simulink model "ICCBF_RVD"  (R2024b)
settings: Solver=ode4  StartTime=0.0  StopTime=tsim  FixedStep=baseRate  RelTol=1e-6  AbsTol=1e-6
values from neighbouring files (symbols this model uses):
  a_KOZ_obs = [0.4, 0.4, 0.4]'    [Run_Initializer.m]
  a_KOZ_tar = [0.4, 0.4, 0.4]'    [Run_Initializer.m]
  a_LOS = [0.4, 0.4, 0.4]'    [Run_Initializer.m]
  beta = pi/2-atan2(docking_offset(1), docking_offset(2))    [Run_Initializer.m]
  docking_offset = [0.165 0.427 -pi/2]'    [Run_Initializer.m]
  eta = sqrt(0.5)    [Run_Initializer.m]
  f = [0 0 0 0 0 0 0]'    [Run_Initializer.m]
  gamma = (0.95)^(baseRate/t_s)    [Run_Initializer.m]
  Gamma1_el = 0.12    [Run_Initializer.m]
  Gamma1_sh = 0.005    [Run_Initializer.m]
  Gamma1_wr = 0.025    [Run_Initializer.m]
  Gamma2_el = 5    [Run_Initializer.m]
  Gamma2_sh = 5    [Run_Initializer.m]
  Gamma2_wr = 5    [Run_Initializer.m]
  Gamma3_el = 10    [Run_Initializer.m]
  Gamma3_sh = 40    [Run_Initializer.m]
  Gamma3_wr = 40    [Run_Initializer.m]
  Gamma4_el = 0.039    [Run_Initializer.m]
  Gamma4_sh = 0.015    [Run_Initializer.m]
  Gamma4_wr = 0.029    [Run_Initializer.m]
  Gamma5_el = 800    [Run_Initializer.m]
  Gamma5_sh = 800    [Run_Initializer.m]
  Gamma5_wr = 800    [Run_Initializer.m]
  Gamma6_el = 0.000001    (= 1e-06)    [Run_Initializer.m]
  Gamma6_sh = 0.005    [Run_Initializer.m]
  Gamma6_wr = 0.02    [Run_Initializer.m]
  H = 2.*diag([1 1 1 p_clf 0 0 0])    [Run_Initializer.m]
  k_dock = 5    [Run_Initializer.m]
  Kd_elarm = 0.8    [Run_Initializer.m]
  Kd_sharm = 1.0    (= 1)    [Run_Initializer.m]
  Kd_wrarm = 0.6    [Run_Initializer.m]
  Kp_elarm = 1.2    [Run_Initializer.m]
  Kp_sharm = 1.5    [Run_Initializer.m]
  Kp_wrarm = 1.0    (= 1)    [Run_Initializer.m]
  PWMFreq = 5    [Run_Initializer.m]
  Q_dock = [(lambda_dock^2)*eye(3) lambda_dock*V ... (first row only)    [Run_Initializer.m]
  r_KOZ_obs = 0.43*[1 1]'    [Run_Initializer.m]
  r_KOZ_tar_min = [0.8; 0.43]    [Run_Initializer.m]
  sensor_FOV = evalin('base', 'sensor_FOV')    [Run_Initializer.m]
  sensor_normal = evalin('base', 'sensor_normal')    [Run_Initializer.m]
  sensor_offset = evalin('base', 'sensor_offset')    [Run_Initializer.m]
  sensor_target = [0.0825 0.2516]'    [Run_Initializer.m]
  tv_CBF = 1    [Run_Initializer.m]
  Tz_lim_elarm = .1    (= 0.1)    [Run_Initializer.m]
  Tz_lim_sharm = .1    (= 0.1)    [Run_Initializer.m]
  Tz_lim_wrarm = .1    (= 0.1)    [Run_Initializer.m]
  u_max = 0.1.*[1 1 (0.3/2)-0.08]'    [Run_Initializer.m]
  x_BLACK_0 = [xLength/2 yLength/2 45*d2r 0 0 1*d2r]'    [Run_Initializer.m]
  x_BLUE_0 = [0 0 0 0 0 0]'    [Run_Initializer.m]
  zeta = 10*d2r    (= 0.174532925199)    [Run_Initializer.m]
undefined symbols (not defined in the file or in its folder): a1, a2, a3, b0, b1, b2, b3, baseRate, dataRate, delta, DiscIntNeverNeededParam, drop_states_ARM, drop_states_BLACK, drop_states_BLUE, drop_states_RED, F_red_X_nominal, F_red_Y_nominal, F_thrusters_BLACK, F_thrusters_BLUE, F_thrusters_RED, home_states_BLACK, home_states_BLUE, home_states_RED, IBLACK, IBLUE, IDIST, IEE, init_states_BLACK, init_states_BLUE, init_states_RED, IPROX, IRED, k1_KOZ_tar, k1_LOS, k2_KOZ_tar, k2_LOS, K_BLACK, K_BLUE, K_RED, k_vel, Kd_tb, Kd_tblue, Kd_tr, Kd_xb, Kd_xblue, Kd_xr, Kd_yb, Kd_yblue, Kd_yr, Kp_tb, Kp_tblue, Kp_tr, Kp_xb, Kp_xblue, Kp_xr, Kp_yb, Kp_yblue, Kp_yr, lambda_KIZ, mBLACK ... (+26)
libraries: simulink x33, nvidiaSharedBlocks x19, dspsigops x7, MainLibrary x4, dspinverses x4
(part 8 of 8)

== matlab function ICCBF_RVD/1 - Experiment Logic/Phase #3: Experiment/Sub-Phase #1/Desired Position RED/Compute Desired Position ==
  data: x_BLACK input; x_des output; docking_offset parameter
function x_des = fcn(x_BLACK, docking_offset)

R = [cos(x_BLACK(3)) -sin(x_BLACK(3)); 
     sin(x_BLACK(3))  cos(x_BLACK(3))];

r_dock = R*(docking_offset(1:2));
x_des = x_BLACK(1:3) + [r_dock; docking_offset(3)];

end

== matlab function ICCBF_RVD/3 - Control/CBF (RED)/Obstacle KOZ CBF ==
  data: x_RED input; A_KOZ_obs output; x_BLUE input; mRED parameter; r_KOZ_obs parameter; b_KOZ_obs output; a_KOZ_obs parameter; IRED parameter; platformSelection parameter
function [A_KOZ_obs, b_KOZ_obs] = fcn(x_RED, x_BLUE, mRED, r_KOZ_obs, a_KOZ_obs, IRED, platformSelection)

if platformSelection >= 6 && platformSelection <= 11
    [g_KOZ_obs, f_KOZ_obs, h_KOZ_obs] = cbf_KOZ(x_RED, x_BLUE, mRED, IRED, r_KOZ_obs, a_KOZ_obs); 
    %A_KOZ_obs = [-g_KOZ_obs, 0, 0, 0, h_KOZ_obs];
    A_KOZ_obs = [-g_KOZ_obs, 0, 0, 0, 0];
    b_KOZ_obs = f_KOZ_obs;
else
    A_KOZ_obs = [0 0 0 0 0 0 0];
    b_KOZ_obs = 0;
end

== matlab function ICCBF_RVD/3 - Control/CBF (RED)/Archives/Target KOZ CBF (OLD) ==
  data: x_RED input; A_KOZ_tar output; x_BLACK input; mRED parameter; r_KOZ_tar input; b_KOZ_tar output; k1_KOZ_tar parameter; k2_KOZ_tar parameter; tv_CBF parameter
function [A_KOZ_tar, b_KOZ_tar] = fcn(x_RED, x_BLACK, mRED, r_KOZ_tar, k1_KOZ_tar, k2_KOZ_tar, tv_CBF)

x_t = x_BLACK(1);
y_t = x_BLACK(2);
theta_t = x_BLACK(3);
x_t_dot = x_BLACK(4);
y_t_dot = x_BLACK(5);
theta_t_dot = x_BLACK(6);

x = x_RED(1);
y = x_RED(2);
x_dot = x_RED(4);
y_dot = x_RED(5);

[a,b] = deal(r_KOZ_tar(1), r_KOZ_tar(2));

A = ((cos(theta_t)/a)^2 + (sin(theta_t)/b)^2);
B = ((sin(theta_t)/a)^2 + (cos(theta_t)/b)^2);
C = 2*sin(theta_t)*cos(theta_t)*(1/a^2-1/b^2);

A_dot = theta_t_dot*sin(2*theta_t)*(b^-2 - a^-2);
B_dot = theta_t_dot*sin(2*theta_t)*(a^-2 - b^-2);
C_dot = 2*theta_t_dot*cos(2*theta_t)*(a^-2 - b^-2);

A_ddot = 2*(theta_t_dot^2)*cos(2*theta_t)*(b^-2 - a^-2);
B_ddot = 2*(theta_t_dot^2)*cos(2*theta_t)*(a^-2 - b^-2);
C_ddot = -4*(theta_t_dot^2)*sin(2*theta_t)*(a^-2 - b^-2);

Lfh = 2*A*(x-x_t)*x_dot + 2*B*(y-y_t)*y_dot + C*(x_dot*(y-y_t) + y_dot*(x-x_t));
Lf2h = 2*A*x_dot^2 + 2*B*y_dot^2 + 2*C*x_dot*y_dot;
LgLfh = [2*A*(x-x_t) + C*(y-y_t), 2*B*(y-y_t) + C*(x-x_t), 0]/mRED;

if tv_CBF == 1
    dhdt = A_dot*(x-x_t)^2 + B_dot*(y-y_t)^2 + C_dot*(x-x_t)*(y-y_t) ...
        - 2*A*(x-x_t)*x_t_dot - 2*B*(y-y_t)*y_t_dot - C*(x_t_dot*(y-y_t)+y_t_dot*(x-x_t));
    ddhddt = A_ddot*(x-x_t)^2 + B_ddot*(y-y_t)^2 + C_ddot*(x-x_t)*(y-y_t) ...
        - 4*A_dot*(x-x_t)*x_t_dot - 4*B_dot*(y-y_t)*y_t_dot ...
        - 2*C_dot*(x_t_dot*(y-y_t) + y_t_dot*(x-x_t)) + 2*A*x_t_dot^2 ...
        + 2*B*y_t_dot^2 + 2*C*x_t_dot*y_t_dot;
    ddtdhdxf = 2*A_dot*(x-x_t)*x_dot - 2*A*x_t_dot*x_dot ...
        + 2*B_dot*(y-y_t)*y_dot - 2*B*y_t_dot*y_dot ...
        + C_dot*(x_dot*(y-y_t) + y_dot*(x-x_t)) - C*(x_t_dot*y_dot + y_t_dot*x_dot);
else
    dhdt = 0;
    ddhddt = 0;
    ddtdhdxf = 0;
end

h = A*(x-x_t)^2 + B*(y-y_t)^2 + C*(x-x_t)*(y-y_t)-1;
h_dot = Lfh + dhdt;

A_KOZ_tar = [-LgLfh 0];
b_KOZ_tar = Lf2h + 2*ddtdhdxf + ddhddt + 2*sqrt(k1_KOZ_tar)*k2_KOZ_tar*h_dot + k1_KOZ_tar*h;

end

== matlab function ICCBF_RVD/3 - Control/CBF (RED)/Archives/Nominal LQR Controller/Calculate Error/MATLAB Function ==
  data: Rz_path input; Rz_error output; Rz_measured input
function Rz_error = SmoothAngularDifference(Rz_path, Rz_measured)

    Rz_error = mod(Rz_measured-Rz_path+pi, 2*pi)-pi;


end

== matlab function ICCBF_RVD/3 - Control/CBF (RED)/Apply CBFs ==
  data: u output; x output; A_KOZ_tar input; b_KOZ_tar input; A_LOS input; b_LOS input; A_KOZ_obs input; b_KOZ_obs input; res output; A_dock input; b_dock input; x0 input; u_max parameter; H parameter; f parameter
function [u, x, res] = fcn(A_KOZ_tar, b_KOZ_tar, A_LOS, b_LOS, A_KOZ_obs, b_KOZ_obs, A_dock, b_dock, x0, u_max, H, f)

A = [A_KOZ_tar; A_LOS; A_KOZ_obs; A_dock];
b = [b_KOZ_tar; b_LOS; b_KOZ_obs; b_dock];

options = optimoptions('quadprog', 'Algorithm', 'active-set', 'MaxIterations', 20);

tic
[x, ~, exitflag, output] = quadprog(H, f, A, b, [], [], [-u_max; 0; 0; 0; 0], [u_max; inf; inf; inf; inf], x0, options);
res = [double(exitflag), double(output.iterations), toc];

u = x(1:3);

end

== matlab function ICCBF_RVD/3 - Control/CBF (RED)/Archives/Velocity CBF (OLD) ==
  data: x_RED input; A_vel output; b_vel output; mRED parameter; k_vel parameter; v_max parameter
function [A_vel, b_vel] = fcn(x_RED, mRED, k_vel, v_max)

x_dot = x_RED(4);
y_dot = x_RED(5);

v_mag = sqrt(x_dot^2+y_dot^2);

Lgh = [(-x_dot/(mRED*v_mag)) (-y_dot/(mRED*v_mag)) 0];
   
h = v_max-v_mag;

A_vel = -Lgh;
b_vel = k_vel*h;

end

== matlab function ICCBF_RVD/Simulate Plant Dynamics/RED and ARM Dynamics/RED Only/Calculated & Store Measured States/Subsystem1/Enabled Subsystem/MATLAB Function ==
  data: y input; dy output; dt input; tau input; ema_prev input; ema output
function [dy, ema] = realtime_derivative_ema(y, dt, tau, ema_prev)
    % Compute smoothed derivative using Exponential Moving Average
    %
    % Inputs:
    %   y        : Current measurement
    %   dt       : Time step
    %   tau      : Time constant for EMA filter (larger = more smoothing)
    %   ema_prev : Previous EMA value
    %
    % Outputs:
    %   dy  : Smoothed derivative estimate
    %   ema : Updated EMA value
    
    % Calculate smoothing factor from time constant
    alpha = 1 - exp(-dt ./ tau);
    
    % Update Exponential Moving Average
    ema = alpha .* y + (1 - alpha) .* ema_prev;
    
    % Compute derivative using finite difference on smoothed values
    dy = (ema - ema_prev) ./ dt;
end

== matlab function ICCBF_RVD/3 - Control/CBF (RED)/Archives/Build Table KIZ CBF ==
  data: x_RED input; A output; b output; delta parameter; mRED parameter; xLength parameter; yLength parameter; lambda_KIZ parameter
function [A, b] = fcn(x_RED, delta, mRED, xLength, yLength, lambda_KIZ)

x = x_RED(1);
x_dot = x_RED(4);

y = x_RED(2);
y_dot = x_RED(5);

h_upper_x = x-delta;
h_dot_upper_x = x_dot;

h_lower_x = -x-delta+xLength;
h_dot_lower_x = -x_dot;

A_upper_x = [-1/mRED 0 0];
b_upper_x = (lambda_KIZ^2)*h_upper_x + 2*lambda_KIZ*h_dot_upper_x;

A_lower_x = [1/mRED 0 0];
b_lower_x = (lambda_KIZ^2)*h_lower_x + 2*lambda_KIZ*h_dot_lower_x;

h_upper_y = y-delta;
h_dot_upper_y = y_dot;

h_lower_y = -y-delta+yLength;
h_dot_lower_y = -y_dot;

A_upper_y = [0 -1/mRED 0];
b_upper_y = (lambda_KIZ^2)*h_upper_y + 2*lambda_KIZ*h_dot_upper_y;

A_lower_y = [0 1/mRED 0];
b_lower_y = (lambda_KIZ^2)*h_lower_y + 2*lambda_KIZ*h_dot_lower_y;

A = [A_upper_x; A_lower_x; A_upper_y; A_lower_y];
b = [b_upper_x; b_lower_x; b_upper_y; b_lower_y];

end

== matlab function ICCBF_RVD/Thruster & Float Control Code/Change BLACK Behavior/Calculate Duty Cycle/Generate Initial Guess/MATLAB Function ==
  data: H output; thruster_dist2CG_BLACK parameter; F_thrusters_BLACK parameter
function H = MakeH(thruster_dist2CG_BLACK,F_thrusters_BLACK)

    Vec1 = [ -1
             -1
              0 
              0
              1
              1
              0
              0 ];
          
    Vec2 = [  0
              0
              1
              1
              0
              0
             -1
             -1 ];
         
    Vec3 = thruster_dist2CG_BLACK./1000;
    
    Mat1 = [Vec1, Vec2, Vec3]';
    
    Mat2 = diag((F_thrusters_BLACK./2));
    
    H    = Mat1*Mat2;

end

== matlab function ICCBF_RVD/Thruster & Float Control Code/Change RED Behavior/Calculate Duty Cycle/MATLAB Function5 ==
  data: H_final output; u_desired input; duty_cycles output; x0 input; thruster_dist2CG_RED parameter; F_red_X_nominal parameter; F_red_Y_nominal parameter; max_iters parameter; tol parameter
function [H_final, duty_cycles] = optimize_duty_cycle_with_decay( ...
    u_desired, x0, thruster_dist2CG_RED, F_red_X_nominal, F_red_Y_nominal, max_iters, tol)
    %OPTIMIZE_DUTY_CYCLE_WITH_DECAY 
    %   Iteratively optimizes thruster duty cycles while updating thrust decay.
    %
    %   Inputs:
    %       u_desired           - Desired force/torque vector [Fx; Fy; M] (3x1)
    %       x0                  - Initial guess for duty cycles (8x1)
    %       thruster_dist2CG_RED- Distances of thrusters from CG (vector, mm)
    %       F_red_X_nominal     - Nominal X-direction thruster force (scalar, N)
    %       F_red_Y_nominal     - Nominal Y-direction thruster force (scalar, N)
    %       max_iters           - Maximum optimization iterations
    %       tol                 - Convergence tolerance (on duty cycles)
    %
    %   Outputs:
    %       H_final     - Final H-matrix including thrust decay (3x8)
    %       duty_cycles - Optimized duty cycles (8x1)
    %

    % ---------------------------
    % Initialization
    % ---------------------------
    num_thrusters      = length(x0); %#ok<NASGU> % reserved if needed later
    duty_cycles        = x0;                     % current solution
    thrust_decay_factor = 1;                     % initial decay
    prev_duty_cycles   = duty_cycles + 2*tol;    % force first iteration

    % ---------------------------
    % Iterative optimization
    % ---------------------------
    for iter = 1:max_iters
        % Build system matrix H with current decay factor
        H = MakeHWithDecay(thruster_dist2CG_RED, F_red_X_nominal, ...
                           thrust_decay_factor, F_red_Y_nominal);

        % Solve constrained least squares (box constraints: 0 ≤ x ≤ 1)
        duty_cycles = custom_constrained_least_squares(H, u_desired, duty_cycles);

        % Update decay factor based on the current duty cycles
        [thrust_decay_factor, ~] = check_thrust_decay(duty_cycles);

        % Check convergence (∞-norm difference)
        if norm(duty_cycles - prev_duty_cycles, Inf) < tol
            H_final = MakeHWithDecayRecalculateForce(thruster_dist2CG_RED, ...
                        F_red_X_nominal, thrust_decay_factor, F_red_Y_nominal);
            return;
        end

        % Update reference for next iteration
        prev_duty_cycles = duty_cycles;
    end

    % If not converged within max_iters, return final H with last decay
    H_final = MakeHWithDecayRecalculateForce(thruster_dist2CG_RED, ...
                F_red_X_nominal, thrust_decay_factor, F_red_Y_nominal);
end


% ========================================================================
% Custom Constrained Least Squares Solver
% ========================================================================
function x_opt = custom_constrained_least_squares(H, b, x0)
    %CUSTOM_CONSTRAINED_LEAST_SQUARES
    %   Solves min_x ||H*x - b||^2 subject to 0 <= x <= 1
    %   using projected gradient descent with backtracking line search.
    %
    %   Inputs:
    %       H   - System matrix (3x8)
    %       b   - Desired vector (3x1)
    %       x0  - Initial guess (8x1)
    %
    %   Output:
    %       x_opt - Optimal duty cycle vector (8x1)

    % Parameters
    max_iterations = 100;
    tolerance      = 1e-6;
    alpha          = 0.01;  % initial step size
    beta           = 0.5;   % backtracking factor

    % Initialization
    x      = x0;
    x_prev = x0 + 2*tolerance;

    % Precompute matrices
    HtH = H' * H;
    Htb = H' * b;

    for iter = 1:max_iterations
        % Gradient of ||H*x - b||^2
        gradient = 2 * (HtH*x - Htb);

        % Store objective for comparison
        current_obj = norm(H*x - b)^2;

        % Backtracking line search
        step_size = alpha;
        for ls_iter = 1:20
            x_new = x - step_size * gradient;
            x_new = max(0, min(1, x_new)); % project into [0,1]

            new_obj = norm(H*x_new - b)^2;
            if new_obj < current_obj
                break; % accept step
            else
                step_size = step_size * beta;
            end
        end

        % Update
        x = x_new;

        % Convergence check
        if norm(x - x_prev) < tolerance
            break;
        end

        % Adaptive step size tuning
        if iter > 1 && new_obj < current_obj
            alpha = min(alpha * 1.1, 0.1); % speed up if progress
        else
            alpha = alpha * 0.9;           % slow down otherwise
        end

        % Store for next iteration
        x_prev = x;
    end

    x_opt = x;
end


% ========================================================================
% Construct H-matrix (with decay factor)
% ========================================================================
function H = MakeHWithDecay(thruster_dist2CG, F_X_nominal, thrust_decay_factor, F_Y_nominal)
    %MAKEHWITHDECAY
    %   Builds the H matrix that maps thruster duty cycles to [Fx; Fy; M],
    %   applying thrust decay.
    %
    %   Outputs H as (3x8)

    % Convert thruster arm distances to meters
    adjusted_dist = thruster_dist2CG / 1000;

    % Thruster directions (X, Y, and moment arm)
    Vec1 = [-1; -1;  0;  0;  1;  1;  0;  0]; % X
    Vec2 = [ 0;  0;  1;  1;  0;  0; -1; -1]; % Y
    Vec3 = adjusted_dist;                    % moment (Z)

    Mat1 = [Vec1, Vec2, Vec3]';

    % Thruster forces (scaled by decay)
    F_thrusters = [F_X_nominal; F_X_nominal; ...
                   F_Y_nominal; F_Y_nominal; ...
                   F_X_nominal; F_X_nominal; ...
                   F_Y_nominal; F_Y_nominal] * thrust_decay_factor;

    % Build diagonal scaling
    Mat2 = diag(F_thrusters / 2);

    % Final mapping
    H = Mat1 * Mat2;
end


% ========================================================================
% Construct H-matrix (recalculate full force with decay)
% ========================================================================
function H = MakeHWithDecayRecalculateForce(thruster_dist2CG, F_X_nominal, thrust_decay_factor, F_Y_nominal)
    %MAKEHWITHDECAYRECALCULATEFORCE
    %   Same as MakeHWithDecay but applies full nominal force scaling.

    adjusted_dist = thruster_dist2CG / 1000;

    Vec1 = [-1; -1;  0;  0;  1;  1;  0;  0];
    Vec2 = [ 0;  0;  1;  1;  0;  0; -1; -1];
    Vec3 = adjusted_dist;

    Mat1 = [Vec1, Vec2, Vec3]';

    F_thrusters = [F_X_nominal; F_X_nominal; ...
                   F_Y_nominal; F_Y_nominal; ...
                   F_X_nominal; F_X_nominal; ...
                   F_Y_nominal; F_Y_nominal] * thrust_decay_factor;

    Mat2 = diag(F_thrusters);

    H = Mat1 * Mat2;
end


% ========================================================================
% Thrust Decay Update Rule
% ========================================================================
function [thrust_decay_factor, count] = check_thrust_decay(PWMs)
    %CHECK_THRUST_DECAY
    %   Updates thrust decay factor based on average duty cycle.
    %
    %   Inputs:
    %       PWMs - Duty cycle vector (8x1)
    %
    %   Outputs:
    %       thrust_decay_factor - Adjusted decay factor (scalar)
    %       count               - Number of active thrusters

    % Normalize if needed
    if max(PWMs) > 1
        PWMs = PWMs / max(PWMs);
    end
    
    % Active thrusters
    count = sum(PWMs > 0);
    
    % Mean duty cycle (only active thrusters)
    avg_duty = sum(max(PWMs, 0)) / max(count, 1);
    
    % Update rule (piecewise)
    if avg_duty < 0.3 || count == 0
        thrust_decay_factor = 1;
    else
        thrust_decay_factor = max(0.6 - 2*avg_duty + 1, 0.5);
    end
end

== matlab function ICCBF_RVD/Thruster & Float Control Code/Change BLACK Behavior/Calculate Duty Cycle/Rotate Forces to Inertial/Create Rotation Matrix ==
  data: Rz input; C_Ib output
function C_Ib = RotateFrame(Rz)

C_bI = [  cos(Rz) sin(Rz)
         -sin(Rz) cos(Rz) ];

C_Ib = inv(C_bI);

end

== matlab function ICCBF_RVD/3 - Control/CBF (RED)/Docking CLF ==
  data: x_RED input; x_BLACK input; A_dock output; b_dock output; mRED parameter; IRED parameter; docking_offset parameter; Q_dock parameter; k_dock parameter; tv_CBF parameter
function [A_dock, b_dock] = fcn(x_RED, x_BLACK, mRED, IRED, docking_offset, Q_dock, k_dock, tv_CBF)

B = [  0       0      0;
       0       0      0;
       0       0      0;
     1/mRED    0      0;
     0      1/mRED    0;
     0         0   1/IRED];

R = [cos(x_BLACK(3)) -sin(x_BLACK(3)); 
     sin(x_BLACK(3))  cos(x_BLACK(3))];
dR = [-sin(x_BLACK(3)) -cos(x_BLACK(3)); 
       cos(x_BLACK(3))  -sin(x_BLACK(3))];

r_des = x_BLACK(1:2) + R*(docking_offset(1:2));
theta_des = wrapAngle(x_BLACK(3) + docking_offset(3));
v_des = x_BLACK(4:5) + x_BLACK(6)*dR*(docking_offset(1:2));
omega_des = x_BLACK(6);

x_des = [r_des; theta_des; v_des; omega_des];

LfV = 2*(x_RED-x_des)'*Q_dock*[x_RED(4:6); 0; 0; 0];
LgV = 2*(x_RED-x_des)'*Q_dock*B;

if tv_CBF == 1
    dVdt = -2*(x_RED-x_des)'*Q_dock*[x_des(4:6); 0; 0; 0];
else
    dVdt = 0;
end

A_dock = [LgV -1 0 0 0];
b_dock = (-LfV - dVdt - k_dock*(x_RED-x_des)'*Q_dock*(x_RED-x_des)); 

end

%% Functions

function theta_wrap = wrapAngle(theta)
    theta_wrap = atan2(sin(theta),cos(theta));
end

== matlab function ICCBF_RVD/Thruster & Float Control Code/Change RED Behavior/Calculate Duty Cycle/MATLAB Function8 ==
  data: ThrustPer_Final output; ThrustPer input; PWMFreq parameter
function ThrustPer_Final  = ThrusterSat(ThrustPer, PWMFreq)

    ValveTime       = 0.007;
    TControl        = 1/PWMFreq;

    ThrustPer_Final = zeros(8,1);
    
    if max(ThrustPer) > 1
        ThrustPer_Sat = ThrustPer/max(ThrustPer);
    else
        ThrustPer_Sat = ThrustPer;
    end
    
    for i = 1:8
        if ThrustPer_Sat(i) > ValveTime/TControl 
            ThrustPer_Final(i) = ThrustPer_Sat(i);
        else
            ThrustPer_Final(i) = 0;
        end
    end


end

== matlab function ICCBF_RVD/Thruster & Float Control Code/Change BLACK Behavior/Rotate Forces to Body/Create Rotation Matrix ==
  data: Rz input; C_bI output
function C_bI = RotateFrame(Rz)

C_bI = [  cos(Rz) sin(Rz)
         -sin(Rz) cos(Rz) ];

end

== matlab function ICCBF_RVD/3 - Control/CBF (RED)/Archives/LOS CBF original (OLD) ==
  data: x_RED input; A_LOS output; x_BLACK input; b_LOS output; k2_LOS parameter; k1_LOS parameter; theta_FOV parameter; IRED parameter; tv_CBF parameter
function [A_LOS, b_LOS] = fcn(x_RED, x_BLACK, k2_LOS, k1_LOS, theta_FOV, IRED, tv_CBF)

x_t = x_BLACK(1);
y_t = x_BLACK(2);
x_t_dot = x_BLACK(4);
y_t_dot = x_BLACK(5);

x = x_RED(1);
y = x_RED(2);
theta = x_RED(3);
x_dot = x_RED(4);
y_dot = x_RED(5);
theta_dot = x_RED(6);
x_ddot = 0;
y_ddot = 0;

theta_star = rotateToFace(x_RED(3), x_BLACK(1:2)-x_RED(1:2));

rmagsq = (x_t-x)^2+(y_t-y)^2;
drmagsqdt = 2*(x_t-x)*(x_t_dot-x_dot)+2*(y_t-y)*(y_t_dot-y_dot);

Lfh = -theta_dot;
LgLfh = [0, 0, -1/IRED];

if tv_CBF == 1
    dh_dt = -((x_t_dot-x_dot)*(y_t-y)-(y_t_dot-y_dot)*(x_t-x))/(rmagsq);
    ddh_dtt = (((y_ddot*(x_t-x)-x_ddot*(y_t-y))*rmagsq) - drmagsqdt*((x_t_dot-x_dot)*(y_t-y)-(y_t_dot-y_dot)*(x_t-x)))/rmagsq^2;
    ddtdhdxf = 0;    
else
    dh_dt = 0;
    ddh_dtt = 0;
    ddtdhdxf = 0;    
end

h_upper = -theta + theta_star + theta_FOV;
h_lower = theta - theta_star + theta_FOV;

h_dot_upper = Lfh + dh_dt;
h_dot_lower = -Lfh - dh_dt;

A_upper = -LgLfh;
A_lower = -(-LgLfh);

b_upper = -2*ddtdhdxf + ddh_dtt + 2*sqrt(k1_LOS)*k2_LOS*h_dot_upper + k1_LOS*h_upper;
b_lower = (-2*ddtdhdxf) + (-ddh_dtt) + 2*sqrt(k1_LOS)*k2_LOS*h_dot_lower + k1_LOS*h_lower;

A_LOS = [A_lower; A_upper];
b_LOS = [b_lower; b_upper];

end

%% Functions

function theta_des = rotateToFace(theta, r)
    theta_des = theta + wrapToPi(atan2(r(2),r(1)) - theta);
end

== matlab function ICCBF_RVD/Thruster & Float Control Code/Change BLUE Behavior/Calculate Duty Cycle/Generate Initial Guess/MATLAB Function ==
  data: H output; thruster_dist2CG_BLUE parameter; F_thrusters_BLUE parameter
function H = MakeH(thruster_dist2CG_BLUE,F_thrusters_BLUE)

    Vec1 = [ -1
             -1
              0 
              0
              1
              1
              0
              0 ];
          
    Vec2 = [  0
              0
              1
              1
              0
              0
             -1
             -1 ];
         
    Vec3 = thruster_dist2CG_BLUE./1000;
    
    Mat1 = [Vec1, Vec2, Vec3]';
    
    Mat2 = diag((F_thrusters_BLUE./2));
    
    H    = Mat1*Mat2;

end

== matlab function ICCBF_RVD/3 - Control/CBF (RED)/Archives/LOS CBF alt (OLD) ==
  data: x_RED input; A_LOS output; x_BLACK input; b_LOS output; k2_LOS parameter; k1_LOS parameter; theta_FOV parameter; IRED parameter; tv_CBF parameter
function [A_LOS, b_LOS] = fcn(x_RED, x_BLACK, k2_LOS, k1_LOS, theta_FOV, IRED, tv_CBF)

x_t = x_BLACK(1);
y_t = x_BLACK(2);
x_t_dot = x_BLACK(4);
y_t_dot = x_BLACK(5);

x = x_RED(1);
y = x_RED(2);
theta = x_RED(3);
theta_dot = x_RED(6);

theta_star = rotateToFace(x_RED(3), x_BLACK(1:2)-x_RED(1:2));

rmagsq = (x_t-x)^2+(y_t-y)^2;

Lfh = -theta_dot;

LgLfh = [0, 0, -1/IRED];

dthetastar_dt = (y_t_dot*(x_t-x) - x_t_dot*(y_t-y))/(rmagsq);
ddthetastar_dt = -2*(((x_t-x)*y_t_dot - (y_t-y)*x_t_dot)*((x_t-x)*x_t_dot+(y_t-y)*y_t_dot))/rmagsq^2;
if tv_CBF == 1
    dh_dt = dthetastar_dt;
    ddh_dtt = ddthetastar_dt;
    ddtdhdxf = 0;    
else
    dh_dt = 0;
    ddh_dtt = 0;
    ddtdhdxf = 0;    
end

h_upper = -theta + theta_star + theta_FOV;
h_lower = theta - theta_star + theta_FOV;

h_dot_upper = Lfh + dh_dt;
h_dot_lower = -Lfh - dh_dt;

A_upper = -LgLfh;
A_lower = -(-LgLfh);

b_upper =  2*ddtdhdxf + ddh_dtt + 2*sqrt(k1_LOS)*k2_LOS*h_dot_upper + k1_LOS*h_upper;
b_lower = (-2*ddtdhdxf) + (-ddh_dtt) + 2*sqrt(k1_LOS)*k2_LOS*h_dot_lower + k1_LOS*h_lower;

A_LOS = [A_lower; A_upper];
b_LOS = [b_lower; b_upper];

end

%% Functions

function theta_des = rotateToFace(theta, r)
    theta_des = theta + wrapToPi(atan2(r(2),r(1)) - theta);
end

== matlab function ICCBF_RVD/Thruster & Float Control Code/Change BLUE Behavior/Calculate Duty Cycle/MATLAB Function1 ==
  data: ThrustPer_Final output; ThrustPer input; PWMFreq parameter
function ThrustPer_Final  = ThrusterSat(ThrustPer, PWMFreq)

    ValveTime       = 0.007;
    TControl        = 1/PWMFreq;

    ThrustPer_Final = zeros(8,1);
    
    if max(ThrustPer) > 1
        ThrustPer_Sat = ThrustPer/max(ThrustPer);
    else
        ThrustPer_Sat = ThrustPer;
    end
    
    for i = 1:8
        if ThrustPer_Sat(i) > ValveTime/TControl 
            ThrustPer_Final(i) = ThrustPer_Sat(i);
        else
            ThrustPer_Final(i) = 0;
        end
    end


end

== matlab function ICCBF_RVD/Thruster & Float Control Code/Change BLUE Behavior/Calculate Duty Cycle/Rotate Forces to Inertial/Create Rotation Matrix ==
  data: Rz input; C_Ib output
function C_Ib = RotateFrame(Rz)

C_bI = [  cos(Rz) sin(Rz)
         -sin(Rz) cos(Rz) ];

C_Ib = inv(C_bI);

end

== matlab function ICCBF_RVD/Thruster & Float Control Code/Change RED Behavior/Calculate Duty Cycle/Rotate Forces to Inertial/Create Rotation Matrix ==
  data: Rz input; C_Ib output
function C_Ib = RotateFrame(Rz)

C_bI = [  cos(Rz) sin(Rz)
         -sin(Rz) cos(Rz) ];

C_Ib = inv(C_bI);

end

== matlab function ICCBF_RVD/Thruster & Float Control Code/Change BLUE Behavior/Rotate Forces to Body/Create Rotation Matrix ==
  data: Rz input; C_bI output
function C_bI = RotateFrame(Rz)

C_bI = [  cos(Rz) sin(Rz)
         -sin(Rz) cos(Rz) ];

end

== matlab function ICCBF_RVD/1 - Experiment Logic/Phase #3: Experiment/Sub-Phase #2/Desired Position BLACK/Safe Desired Position ==
  data: x_des input; x_des output; x_des_prev input; xLength parameter; yLength parameter
function x_des = fcn(x_des,x_des_prev, xLength, yLength)

corners = [0 0;
           xLength 0;
           xLength yLength;
           0 yLength];

walls = [ 1  0;
          0  1;
         -1  0;
          0 -1];

edge = 0;
for j = 1:length(walls)
    wall_normal = [-walls(j,2); walls(j,1)];

    if dot(x_des(4:5), -wall_normal) > 0
        % Not moving towards wall
        continue
    end

    d = norm(dot(x_des(1:2) - corners(j,:)', wall_normal))/norm(walls(j,:)');
    if d <= 0.3
        edge = 1;
        break
    end
end

if edge
    x_des = x_des_prev;
end

== matlab function ICCBF_RVD/1 - Experiment Logic/Phase #3: Experiment/Sub-Phase #2/Desired Position BLUE/Safe Desired Position ==
  data: x_des input; x_des output; x_des_prev input; xLength parameter; yLength parameter
function x_des = fcn(x_des,x_des_prev, xLength, yLength)

corners = [0 0;
           xLength 0;
           xLength yLength;
           0 yLength];

walls = [ 1  0;
          0  1;
         -1  0;
          0 -1];

edge = 0;
for j = 1:length(walls)
    wall_normal = [-walls(j,2); walls(j,1)];

    if dot(x_des(4:5), -wall_normal) > 0
        % Not moving towards wall
        continue
    end

    d = norm(dot(x_des(1:2) - corners(j,:)', wall_normal))/norm(walls(j,:)');
    if d <= 0.3
        edge = 1;
        break
    end
end

if edge
    x_des = x_des_prev;
end

== matlab function ICCBF_RVD/3 - Control/CBF (RED)/Target KOZ ICCBF ==
  data: x_RED input; A_KOZ_tar output; x_BLACK input; mRED parameter; IRED parameter; b_KOZ_tar output; a_KOZ_tar parameter; r_KOZ_tar input
function [A_KOZ_tar, b_KOZ_tar] = fcn(x_RED, x_BLACK, mRED, IRED, a_KOZ_tar, r_KOZ_tar)

[g_KOZ_tar, f_KOZ_tar, h_KOZ_tar] = cbf_KOZ(x_RED, x_BLACK, mRED, IRED, r_KOZ_tar, a_KOZ_tar);

%A_KOZ_tar = [-g_KOZ_tar, 0, h_KOZ_tar, 0, 0];
A_KOZ_tar = [-g_KOZ_tar, 0, 0, 0, 0];
b_KOZ_tar = f_KOZ_tar;

end

== matlab function ICCBF_RVD/Thruster & Float Control Code/Change RED Behavior/Rotate Forces to Body/Create Rotation Matrix ==
  data: Rz input; C_bI output
function C_bI = RotateFrame(Rz)

C_bI = [  cos(Rz) sin(Rz)
         -sin(Rz) cos(Rz) ];

end

== matlab function ICCBF_RVD/1 - Experiment Logic/Phase #3: Experiment/Sub-Phase #2/Desired Position RED/Compute Desired Position ==
  data: x_BLACK input; x_des output; docking_offset parameter
function x_des = fcn(x_BLACK, docking_offset)

R = [cos(x_BLACK(3)) -sin(x_BLACK(3)); 
     sin(x_BLACK(3))  cos(x_BLACK(3))];

r_dock = R*(docking_offset(1:2));
x_des = x_BLACK(1:3) + [r_dock; docking_offset(3)];

end

== matlab function ICCBF_RVD/3 - Control/CBF (RED)/Clamp to u_max ==
  data: u input; u output; u_max parameter
function u = fcn(u, u_max)

if abs(u(1)) > u_max(1)
    u(1) = sign(u(1))*u_max(1);
end 

if abs(u(2)) > u_max(2)
    u(2) = sign(u(2))*u_max(2);
end 

if abs(u(3)) > u_max(3)
    u(3) = sign(u(3))*u_max(3);
end

end

== matlab function ICCBF_RVD/3 - Control/Default LQR Control (RED)/Calculate Error/MATLAB Function ==
  data: Rz_path input; Rz_error output; Rz_measured input
function Rz_error = SmoothAngularDifference(Rz_path, Rz_measured)

    Rz_error = mod(Rz_measured-Rz_path+pi, 2*pi)-pi;


end

== matlab function ICCBF_RVD/1 - Experiment Logic/Phase #3: Experiment/Sub-Phase #1/Desired Position BLUE/Safe Desired Position ==
  data: x_des input; x_des output; x_des_prev input; xLength parameter; yLength parameter
function x_des = fcn(x_des,x_des_prev, xLength, yLength)

corners = [0 0;
           xLength 0;
           xLength yLength;
           0 yLength];

walls = [ 1  0;
          0  1;
         -1  0;
          0 -1];

edge = 0;
for j = 1:length(walls)
    wall_normal = [-walls(j,2); walls(j,1)];

    if dot(x_des(1:2)-x_des_prev(1:2), wall_normal) > 0
        % Not moving towards wall
        continue
    end

    d = norm(dot(x_des(1:2) - corners(j,:)', wall_normal))/norm(walls(j,:)');
    if d <= 0.3
        edge = 1;
        break
    end
end

if edge
    x_des = x_des_prev;
end

== matlab function ICCBF_RVD/1 - Experiment Logic/Phase #3: Experiment/Sub-Phase #1/Desired Position BLACK/Safe Desired Position ==
  data: x_des input; x_des output; x_des_prev input; xLength parameter; yLength parameter
function x_des = fcn(x_des,x_des_prev, xLength, yLength)

corners = [0 0;
           xLength 0;
           xLength yLength;
           0 yLength];

walls = [ 1  0;
          0  1;
         -1  0;
          0 -1];

edge = 0;
for j = 1:length(walls)
    wall_normal = [-walls(j,2); walls(j,1)];

    if dot(x_des(1:2)-x_des_prev(1:2), wall_normal) > 0
        % Not moving towards wall
        continue
    end

    d = norm(dot(x_des(1:2) - corners(j,:)', wall_normal))/norm(walls(j,:)');
    if d <= 0.3
        edge = 1;
        break
    end
end

if edge
    x_des = x_des_prev;
end

== matlab function ICCBF_RVD/1 - Experiment Logic/Phase #3: Experiment/Sub-Phase #3/Desired Position BLACK/Safe Desired Position ==
  data: x_des input; x_des output; x_des_prev input; xLength parameter; yLength parameter
function x_des = fcn(x_des,x_des_prev, xLength, yLength)

corners = [0 0;
           xLength 0;
           xLength yLength;
           0 yLength];

walls = [ 1  0;
          0  1;
         -1  0;
          0 -1];

edge = 0;
for j = 1:length(walls)
    wall_normal = [-walls(j,2); walls(j,1)];

    if dot(x_des(4:5), -wall_normal) > 0
        % Not moving towards wall
        continue
    end

    d = norm(dot(x_des(1:2) - corners(j,:)', wall_normal))/norm(walls(j,:)');
    if d <= 0.3
        edge = 1;
        break
    end
end

if edge
    x_des = x_des_prev;
end

== matlab function ICCBF_RVD/1 - Experiment Logic/Phase #3: Experiment/Sub-Phase #3/Desired Position BLUE/Safe Desired Position ==
  data: x_des input; x_des output; x_des_prev input; xLength parameter; yLength parameter
function x_des = fcn(x_des,x_des_prev, xLength, yLength)

corners = [0 0;
           xLength 0;
           xLength yLength;
           0 yLength];

walls = [ 1  0;
          0  1;
         -1  0;
          0 -1];

edge = 0;
for j = 1:length(walls)
    wall_normal = [-walls(j,2); walls(j,1)];

    if dot(x_des(4:5), -wall_normal) > 0
        % Not moving towards wall
        continue
    end

    d = norm(dot(x_des(1:2) - corners(j,:)', wall_normal))/norm(walls(j,:)');
    if d <= 0.3
        edge = 1;
        break
    end
end

if edge
    x_des = x_des_prev;
end

== matlab function ICCBF_RVD/1 - Experiment Logic/Phase #3: Experiment/Sub-Phase #3/Desired Position RED/Compute Desired Position ==
  data: x_BLACK input; x_des output; docking_offset parameter
function x_des = fcn(x_BLACK, docking_offset)

R = [cos(x_BLACK(3)) -sin(x_BLACK(3)); 
     sin(x_BLACK(3))  cos(x_BLACK(3))];

r_dock = R*(docking_offset(1:2));
x_des = x_BLACK(1:3) + [r_dock; docking_offset(3)];

end

== matlab function ICCBF_RVD/Thruster & Float Control Code/Change BLACK Behavior/Calculate Duty Cycle/MATLAB Function1 ==
  data: ThrustPer_Final output; ThrustPer input; PWMFreq parameter
function ThrustPer_Final  = ThrusterSat(ThrustPer, PWMFreq)

    ValveTime       = 0.007;
    TControl        = 1/PWMFreq;

    ThrustPer_Final = zeros(8,1);
    
    if max(ThrustPer) > 1
        ThrustPer_Sat = ThrustPer/max(ThrustPer);
    else
        ThrustPer_Sat = ThrustPer;
    end
    
    for i = 1:8
        if ThrustPer_Sat(i) > ValveTime/TControl 
            ThrustPer_Final(i) = ThrustPer_Sat(i);
        else
            ThrustPer_Final(i) = 0;
        end
    end


end

== matlab function ICCBF_RVD/1 - Experiment Logic/Phase #3: Experiment/Sub-Phase #4/Desired Position BLACK/Safe Desired Position ==
  data: x_des input; x_des output; x_des_prev input; xLength parameter; yLength parameter
function x_des = fcn(x_des,x_des_prev, xLength, yLength)

corners = [0 0;
           xLength 0;
           xLength yLength;
           0 yLength];

walls = [ 1  0;
          0  1;
         -1  0;
          0 -1];

edge = 0;
for j = 1:length(walls)
    wall_normal = [-walls(j,2); walls(j,1)];

    if dot(x_des(4:5), -wall_normal) > 0
        % Not moving towards wall
        continue
    end

    d = norm(dot(x_des(1:2) - corners(j,:)', wall_normal))/norm(walls(j,:)');
    if d <= 0.3
        edge = 1;
        break
    end
end

if edge
    x_des = x_des_prev;
end

== matlab function ICCBF_RVD/1 - Experiment Logic/Phase #3: Experiment/Sub-Phase #4/Desired Position BLUE/Safe Desired Position ==
  data: x_des input; x_des output; x_des_prev input; xLength parameter; yLength parameter
function x_des = fcn(x_des,x_des_prev, xLength, yLength)

corners = [0 0;
           xLength 0;
           xLength yLength;
           0 yLength];

walls = [ 1  0;
          0  1;
         -1  0;
          0 -1];

edge = 0;
for j = 1:length(walls)
    wall_normal = [-walls(j,2); walls(j,1)];

    if dot(x_des(4:5), -wall_normal) > 0
        % Not moving towards wall
        continue
    end

    d = norm(dot(x_des(1:2) - corners(j,:)', wall_normal))/norm(walls(j,:)');
    if d <= 0.3
        edge = 1;
        break
    end
end

if edge
    x_des = x_des_prev;
end

== matlab function ICCBF_RVD/3 - Control/Default LQR Control (BLACK)/Calculate Error/MATLAB Function ==
  data: Rz_path input; Rz_error output; Rz_measured input
function Rz_error = SmoothAngularDifference(Rz_path, Rz_measured)

    Rz_error = mod(Rz_measured-Rz_path+pi, 2*pi)-pi;


end

== matlab function ICCBF_RVD/1 - Experiment Logic/Phase #3: Experiment/Sub-Phase #4/Desired Position RED/Compute Desired Position ==
  data: x_BLACK input; x_des output; docking_offset parameter
function x_des = fcn(x_BLACK, docking_offset)

R = [cos(x_BLACK(3)) -sin(x_BLACK(3)); 
     sin(x_BLACK(3))  cos(x_BLACK(3))];

r_dock = R*(docking_offset(1:2));
x_des = x_BLACK(1:3) + [r_dock; docking_offset(3)];

end

== matlab function ICCBF_RVD/Simulate Plant Dynamics/RED and ARM Dynamics/RED + ARM/Dynamics Model ==
  data: q_dot output; x input; InertiaS input; CoriolisS input; u input; Gamma1_sh parameter; Gamma2_sh parameter; Gamma3_sh parameter; Gamma5_sh parameter; Gamma4_sh parameter; Gamma6_sh parameter; Gamma1_el parameter; Gamma2_el parameter; Gamma3_el parameter; Gamma5_el parameter; Gamma4_el parameter; Gamma6_el parameter; Gamma1_wr parameter; Gamma2_wr parameter; Gamma3_wr parameter; Gamma5_wr parameter; Gamma4_wr parameter; Gamma6_wr parameter; q_ddot output
function [q_dot, q_ddot]  = DynamicsModel(x, InertiaS, CoriolisS, u,...
    Gamma1_sh, Gamma2_sh, Gamma3_sh, Gamma5_sh, Gamma4_sh, Gamma6_sh,...
    Gamma1_el, Gamma2_el, Gamma3_el, Gamma5_el, Gamma4_el, Gamma6_el,...
    Gamma1_wr, Gamma2_wr, Gamma3_wr, Gamma5_wr, Gamma4_wr, Gamma6_wr)


    fqdot1 = Gamma1_sh*(tanh(Gamma2_sh*x(10)) - tanh(Gamma3_sh*x(10))) + Gamma4_sh*tanh(Gamma5_sh*x(10)) + Gamma6_sh*x(10);

    fqdot2 = Gamma1_el*(tanh(Gamma2_el*x(11)) - tanh(Gamma3_el*x(11))) + Gamma4_el*tanh(Gamma5_el*x(11)) + Gamma6_el*x(11);

    fqdot3 = Gamma1_wr*(tanh(Gamma2_wr*x(12)) - tanh(Gamma3_wr*x(12))) + Gamma4_wr*tanh(Gamma5_wr*x(12)) + Gamma6_wr*x(12);
    
    q_dot  = x(7:12);
    q_ddot = pinv(InertiaS)*(u - CoriolisS*x(7:12) - [0;0;0;fqdot1;fqdot2;fqdot3]);
    
end

== matlab function ICCBF_RVD/3 - Control/Default PD Control (RED)/Calculate Error/MATLAB Function ==
  data: Rz_path input; Rz_error output; Rz_measured input
function Rz_error = SmoothAngularDifference(Rz_path, Rz_measured)

    Rz_error = mod(Rz_measured-Rz_path+pi, 2*pi)-pi;


end

== matlab function ICCBF_RVD/3 - Control/Default PD Control (BLACK)/Calculate Error/MATLAB Function ==
  data: Rz_path input; Rz_error output; Rz_measured input
function Rz_error = SmoothAngularDifference(Rz_path, Rz_measured)

    Rz_error = mod(Rz_measured-Rz_path+pi, 2*pi)-pi;


end
